simulink model "HaterL2"  (R2015b)
settings: Solver=ode3  StartTime=0.0  StopTime=inf  FixedStep=0.05  RelTol=1e-3
libraries: robotlib x7
settings Model: Creator=einar  LastModifiedBy=einar
settings OptimizationCC: OptimizeModelRefInitCode=on  LifeSpan=Inf  MaxStackSize=64
settings HardwareCC: ProdBitPerPointer=32  ProdLargestAtomicFloat=None  ProdIntDivRoundTo=Undefined  ProdEndianess=Unspecified  ProdWordSize=32  ProdHWDeviceType=Generic->Unspecified (assume 32-bit Generic)
settings RTWCC: SystemTargetFile=ert.tlc  TemplateMakefile=ert_default_tmf  Description=Embedded Coder  Toolchain=Catkin  TargetLang=C++
settings CodeAppCC: IgnoreCustomStorageClasses=off
settings ERTTargetCC: SupportContinuousTime=on

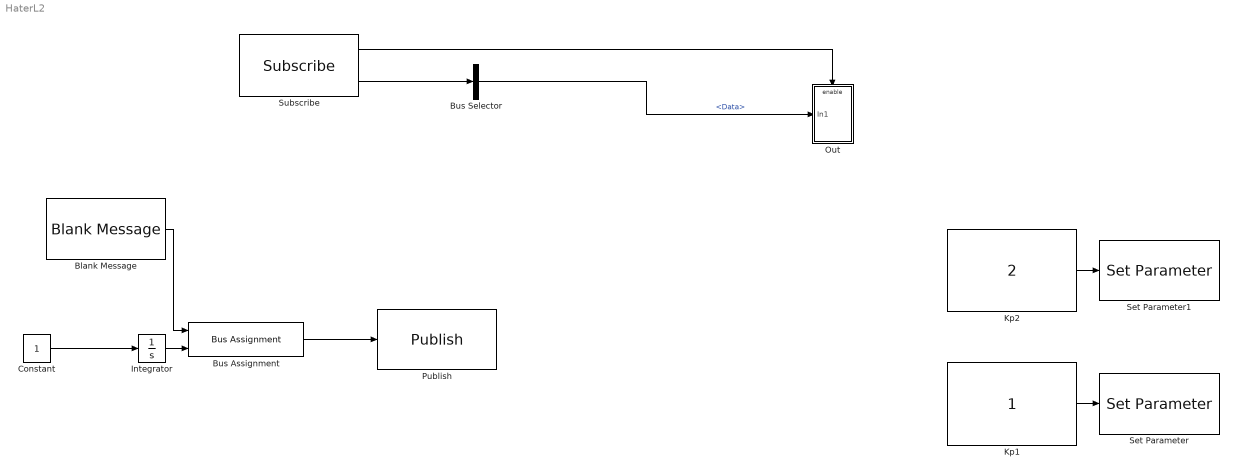
== system HaterL2 ==
  Blank Message : robotlib/Blank Message  SourceLibraryInfo=This block requires Robotics System Toolbox  messageType=std_msgs/Float64  SampleTime=inf
  Bus Assignment : BusAssignment  AssignedSignals=Data
  Bus Selector : BusSelector  OutputSignals=Data
  Constant : Constant
  Integrator : Integrator
  Kp1 : Constant
  Kp2 : Constant  Value=2
  Out : Subsystem
  Publish : robotlib/Publish  SourceLibraryInfo=This block requires Robotics System Toolbox  topicSource=Specify your own  topic=/SimuTime  messageType=std_msgs/Float64  messageQueueLength=1
  Set Parameter : robotlib/Set Parameter  SourceLibraryInfo=This block requires Robotics System Toolbox  ParameterSource=Specify your own  ParameterName=/my_param  ParameterType=double  ModelName=HaterL  BlockId=ParamSet_HaterL_16
  Set Parameter1 : robotlib/Set Parameter  SourceLibraryInfo=This block requires Robotics System Toolbox  ParameterSource=Specify your own  ParameterName=/my_param2  ParameterType=double  ModelName=HaterL  BlockId=ParamSet_HaterL_19
  Subscribe : robotlib/Subscribe  SourceLibraryInfo=This block requires Robotics System Toolbox  topicSource=Specify your own  topic=/PrefPosition  messageType=std_msgs/Float64  sampleTime=-1  messageQueueLength=1
  wires:
  Subscribe/2 -> Bus Selector/1
  Bus Selector/1 -> Out/1(In1)  "<Data>"
  Subscribe/1 -> Out/Enable
  Constant/1 -> Integrator/1
  Bus Assignment/1 -> Publish/1
  Blank Message/1 -> Bus Assignment/1
  Integrator/1 -> Bus Assignment/2
  Kp1/1 -> Set Parameter/1
  Kp2/1 -> Set Parameter1/1

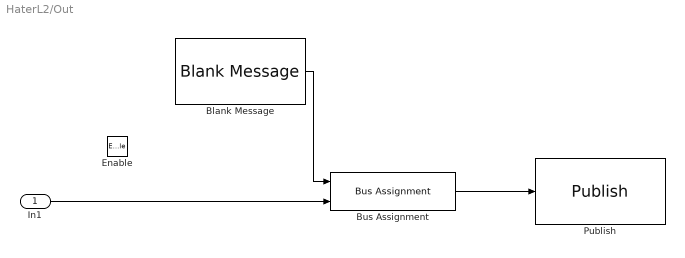
== system HaterL2/Out ==
  In1 : Inport
  Enable : EnablePort
  Blank Message : robotlib/Blank Message  SourceLibraryInfo=This block requires Robotics System Toolbox  messageType=std_msgs/Float64  SampleTime=inf
  Bus Assignment : BusAssignment  AssignedSignals=Data
  Publish : robotlib/Publish  SourceLibraryInfo=This block requires Robotics System Toolbox  topicSource=Specify your own  topic=/PWM  messageType=std_msgs/Float64  messageQueueLength=1
  wires:
  Bus Assignment/1 -> Publish/1
  Blank Message/1 -> Bus Assignment/1
  In1/1 -> Bus Assignment/2
